simulink subsystem "Subsistema_sensor"  (R2023b)
settings: Solver=VariableStepAuto  StartTime=0.0  StopTime=10.0  RelTol=1e-3
libraries: arduinolib x2
settings Model: Creator=manu_  LastModifiedBy=manu_
settings OptimizationCC: ReuseModelBlockBuffer=off

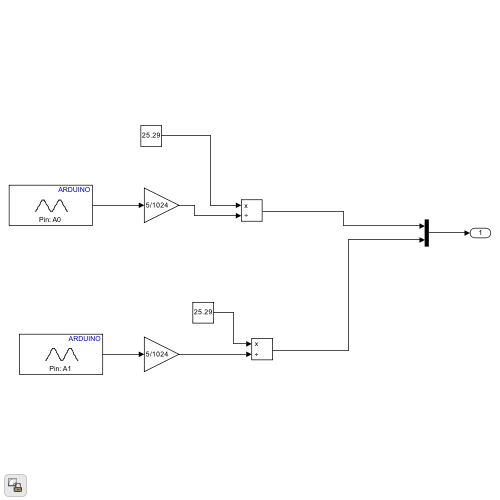
[thumbnail: Simulink's stored preview of the top-level diagram]
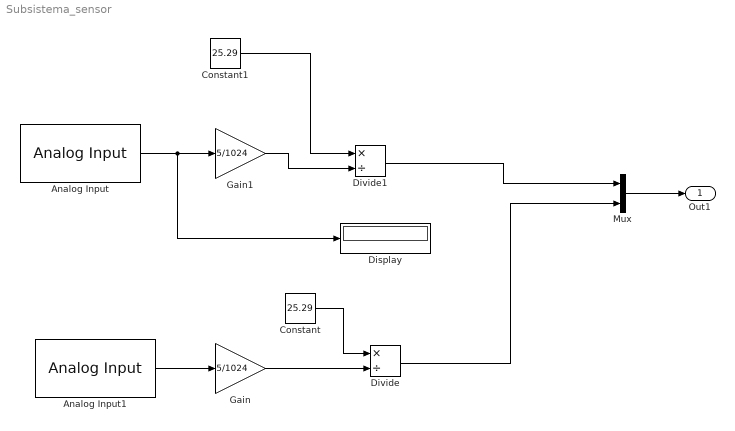
== system Subsistema_sensor ==
  Analog Input : arduinolib/Analog Input  pinNumber=3  ReadResultsOnly=off  ConversionTriggerSource=Software  ExternalTriggerType=uint32( 0 )  OutputDataType=uint16  EnableConversionCompleteNotify=off  EnableOuputStatus=off  SampleTime=-1  blockPlatform=arduino
  Analog Input1 : arduinolib/Analog Input  pinNumber=4  ReadResultsOnly=off  ConversionTriggerSource=Software  ExternalTriggerType=uint32( 0 )  OutputDataType=uint16  EnableConversionCompleteNotify=off  EnableOuputStatus=off  SampleTime=-1  blockPlatform=arduino
  Constant : Constant  Value=25.29
  Constant1 : Constant  Value=25.29
  Display : Display
  Divide : Product  Inputs=*/
  Divide1 : Product  Inputs=*/
  Gain : Gain  Gain=5/1024
  Gain1 : Gain  Gain=5/1024
  Mux : Mux  Inputs=2
  Out1 : Outport
  wires:
  Analog Input/1 -> Gain1/1, Display/1
  Analog Input1/1 -> Gain/1
  Gain/1 -> Divide/2
  Constant/1 -> Divide/1
  Divide/1 -> Mux/2
  Divide1/1 -> Mux/1
  Constant1/1 -> Divide1/1
  Gain1/1 -> Divide1/2
  Mux/1 -> Out1/1
